simulink library "discreteWrapper"  (R2022a)
settings: Solver=VariableStepAuto  StartTime=0.0  StopTime=10.0  RelTol=1e-3
undefined symbols (not defined in the file or in its folder): FLIGHTCONTROLLER, initializeBussesFromBlock, vhcl
libraries: pathFollowingCtrlAoATurbCoefDiscrete_cl x1
settings Model: Creator=adabney  LastModifiedBy=adabney
settings SolverCC: AlgebraicLoopSolver=TrustRegion
settings DebuggingCC: UnconnectedInputMsg=warning  UnconnectedOutputMsg=warning  UnconnectedLineMsg=warning  SFMachineParentedDataDiag=warning

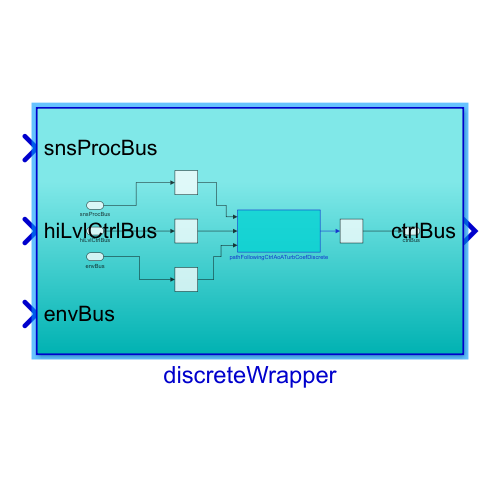
[thumbnail: Simulink's stored preview of the top-level diagram]
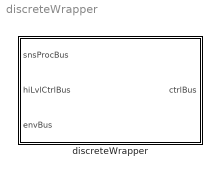
== system discreteWrapper ==
  discreteWrapper : Subsystem  InitFcn=initializeBussesFromBlock(gcb)

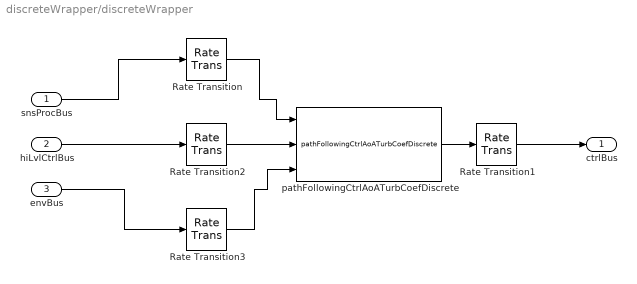
== system discreteWrapper/discreteWrapper ==
  snsProcBus : Inport
  hiLvlCtrlBus : Inport  Port=2
  envBus : Inport  Port=3
  Rate Transition : RateTransition  OutPortSampleTime=fltCtrl.Ts.Value
  Rate Transition1 : RateTransition
  Rate Transition2 : RateTransition  OutPortSampleTime=fltCtrl.Ts.Value
  Rate Transition3 : RateTransition  OutPortSampleTime=fltCtrl.Ts.Value
  pathFollowingCtrlAoATurbCoefDiscrete : pathFollowingCtrlAoATurbCoefDiscrete_cl/pathFollowingCtrlAoATurbCoefDiscrete  VariantControl=strcmpi(FLIGHTCONTROLLER,'pathFollowingControllerManta')  initPosForInitSStar=vhcl.initPosVecGnd.Value  fluidDensity=env.water.density.Value  pathCtrl=pthCtrl1  aeroStruct=vhcl.struct('OCT.aeroSurf')
  ctrlBus : Outport
  wires:
  pathFollowingCtrlAoATurbCoefDiscrete/1 -> Rate Transition1/1
  Rate Transition/1 -> pathFollowingCtrlAoATurbCoefDiscrete/1
  Rate Transition3/1 -> pathFollowingCtrlAoATurbCoefDiscrete/3
  Rate Transition2/1 -> pathFollowingCtrlAoATurbCoefDiscrete/2
  Rate Transition1/1 -> ctrlBus/1
  hiLvlCtrlBus/1 -> Rate Transition2/1
  snsProcBus/1 -> Rate Transition/1
  envBus/1 -> Rate Transition3/1
